simulink model "Model_statespacesystem"  (R2024b)
settings: Solver=ode45  StartTime=0.0  StopTime=30  RelTol=1e-3
values from neighbouring files (symbols this model uses):
  A_o = A_22 - L_obs*A_12    [Controller_StateSpace_Lab1.m]
  B_o = [B_2-L_obs*B_1, (A_22-L_obs*A_12)*L_obs + A_21-L_obs*A_11]    [Controller_StateSpace_Lab1.m]
  C_o = T*[0;1]    [Controller_StateSpace_Lab1.m]
  D_o = T*[0,1;0,L_obs]    [Controller_StateSpace_Lab1.m]
settings Model: Creator=Riccardo Grosso  LastModifiedBy=Buton
settings DataIOCC: ReturnWorkspaceOutputs=off
settings DebuggingCC: AlgebraicLoopMsg=none

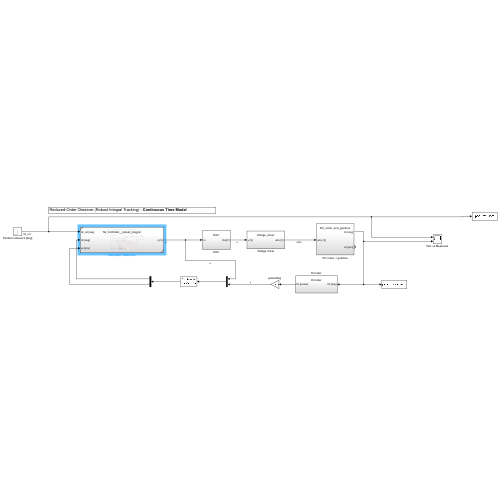
[thumbnail: Simulink's stored preview of the top-level diagram]
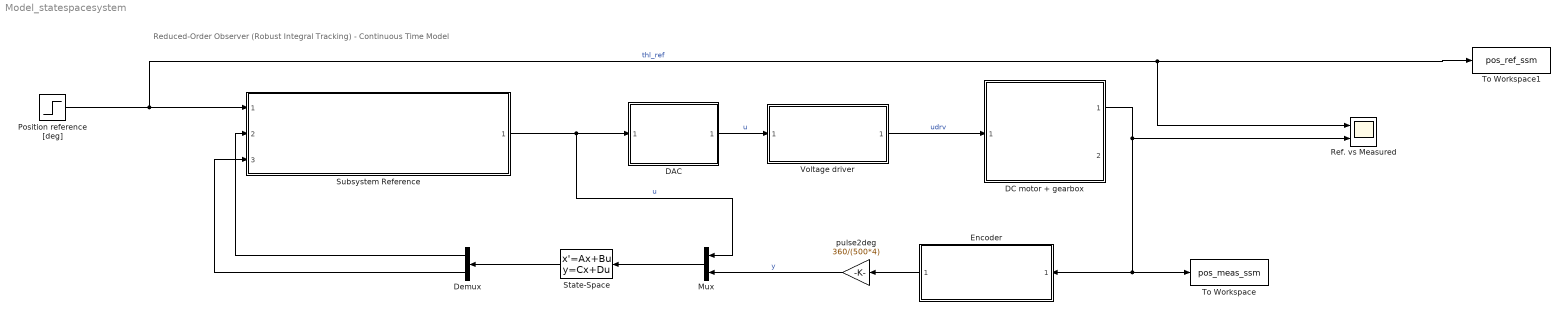
== system Model_statespacesystem ==
  note: Reduced-Order Observer (Robust Integral Tracking) - Continuous Time Model
  DAC : Subsystem  ReferencedSubsystem=DAC
  DC motor + gearbox : Subsystem  ReferencedSubsystem=DC_motor_and_gearbox
  Demux : Demux  Outputs=2
  Encoder : Subsystem  ReferencedSubsystem=Encoder
  Mux : Mux  Inputs=2
  Position reference [deg] : Step  Time=0  After=120  SampleTime=0
  Ref. vs Measured : Scope  NumInputPorts=2
  State-Space : StateSpace  A=A_o  B=B_o  C=C_o  D=D_o  InitialCondition=0
  Subsystem Reference : Subsystem  ReferencedSubsystem=Ss_controller__robust_integral
  To Workspace : ToWorkspace  VariableName=pos_meas_ssm  SaveFormat=Timeseries  SampleTime=-1
  To Workspace1 : ToWorkspace  VariableName=pos_ref_ssm  SaveFormat=Timeseries  SampleTime=-1
  Voltage driver : Subsystem  ReferencedSubsystem=Voltage_driver
  pulse2deg : Gain  Gain=360/(500*4)
  wires:
  DAC/1 -> Voltage driver/1  "u"
  Voltage driver/1 -> DC motor + gearbox/1  "udrv"
  Encoder/1 -> pulse2deg/1
  DC motor + gearbox/1 -> Encoder/1, To Workspace/1, Ref. vs Measured/2
  Position reference [deg]/1 -> Subsystem Reference/1, To Workspace1/1, Ref. vs Measured/1  "thl_ref"
  Subsystem Reference/1 -> Mux/1, DAC/1  "u"
  Mux/1 -> State-Space/1
  pulse2deg/1 -> Mux/2  "y"
  Demux/1 -> Subsystem Reference/2
  Demux/2 -> Subsystem Reference/3
  State-Space/1 -> Demux/1
